simulink model "Linearisierung3_Robo_Sim_9b"  (R2017a)
settings: Solver=VariableStepAuto  StartTime=0.0  StopTime=10.0  RelTol=1e-3
values from neighbouring files (symbols this model uses):
  c = 1    [Linearisierung3_Robo.m]
  g = 9.81    [Linearisierung3_Robo.m]
  l = 1    [Linearisierung3_Robo.m]
  m = 7    [Linearisierung3_Robo.m]
settings Model: Creator=Jonas  LastModifiedBy=jonas

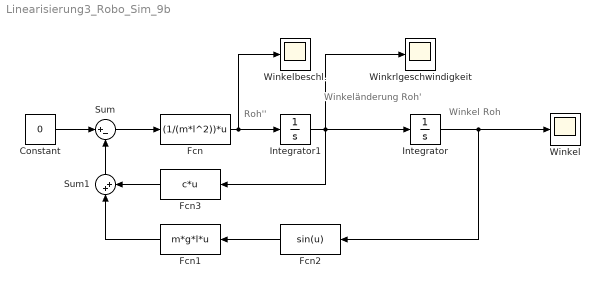
== system Linearisierung3_Robo_Sim_9b ==
  note: Roh''
  note: Winkeländerung
      | Roh'
  note: Winkel Roh
  Constant : Constant  Value=0
  Fcn : Fcn  Expr=(1/(m*l^2))*u
  Fcn1 : Fcn  Expr=m*g*l*u
  Fcn2 : Fcn  Expr=sin(u)
  Fcn3 : Fcn  Expr=c*u
  Integrator : Integrator  InitialCondition=0.6981
  Integrator1 : Integrator
  Sum : Sum  Inputs=|+-
  Sum1 : Sum  Inputs=|++
  "Winkel " : Scope
  Winkelbeschl. : Scope
  "Winkrlgeschwindigkeit " : Scope
  wires:
  Sum1/1 -> Sum/2
  Constant/1 -> Sum/1
  Sum/1 -> Fcn/1
  Fcn3/1 -> Sum1/2
  Fcn1/1 -> Sum1/1
  Fcn2/1 -> Fcn1/1
  Integrator/1 -> "Winkel "/1, Fcn2/1
  Integrator1/1 -> "Winkrlgeschwindigkeit "/1, Fcn3/1, Integrator/1
  Fcn/1 -> Integrator1/1, Winkelbeschl./1
